simulink model "TremorStabilizingSimulation"  (Simulink 10.0)
settings: Solver=ode45  StartTime=0.0  StopTime=500  RelTol=1e-8  EnableMultiTasking=on
PreLoadFcn:
  | % Motor Parameters
  | 
  | J=0.01;     %kg*m^2
  | b=0.1;      %N*m/(rad/s)
  | K=0.01;     %V/(rad/s)
  | R=1;        %Ohm
  | L=0.5;      %H
libraries: simulink_extras x2, simulink x1
settings Model: Creator=deastman  LastModifiedBy=Aarranon
settings DataIOCC: LimitDataPoints=on  SignalLoggingSaveFormat=ModelDataLogs
settings OptimizationCC: ExpressionDepthLimit=2147483647  InitFltsAndDblsToZero=on
settings DebuggingCC: SolverPrmCheckMsg=warning  FcnCallInpInsideContextMsg=warning  StateNameClashWarn=warning
settings GRTTargetCC: GeneratePreprocessorConditionals=Disable all
settings ConfigComp: CovExternalEMLEnable=off

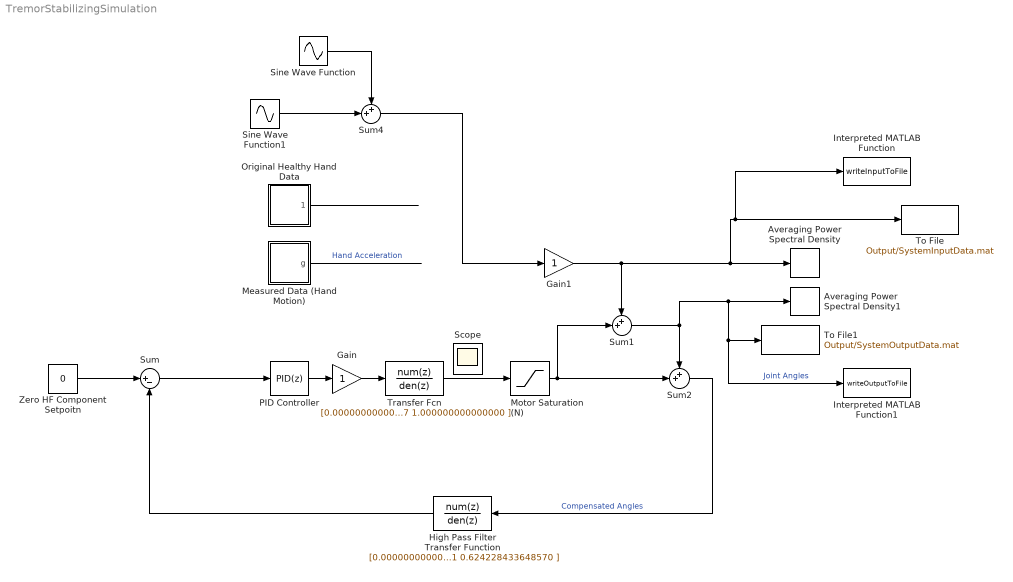
== system TremorStabilizingSimulation ==
  Averaging Power Spectral Density : simulink_extras/Additional Sinks/Averaging Power Spectral Density  npts=128  fftpts=512  HowOften=64  sampleT=2*1/104
      settings: SourceProductName=Simulink  SourceProductBaseCode=SL
  Averaging Power Spectral Density1 : simulink_extras/Additional Sinks/Averaging Power Spectral Density  npts=128  fftpts=512  HowOften=64  sampleT=2*1/104
      settings: SourceProductName=Simulink  SourceProductBaseCode=SL
  Gain : Gain
  Gain1 : Gain
  High Pass Filter Transfer Function : DiscreteTransferFcn  Numerator=[0.000000000000000 0.007900812829378 -0.007900812829378 ]  Denominator=[1.000000000000000 -1.580162565875511 0.624228433648570 ]  SampleTime=0.0100000000000000002  mask(DiscretizedDiscreteTransferFcn){}
      mask init:
      | %zoh
  Interpreted MATLAB Function : MATLABFcn  MATLABFcn=writeInputToFile  OutputDimensions=0
  Interpreted MATLAB Function1 : MATLABFcn  MATLABFcn=writeOutputToFile  OutputDimensions=0
  Measured Data (Hand Motion) : Subsystem
  Motor Saturation (N) : Saturate  UpperLimit=5.5/0.46  LowerLimit=-5.5/0.46
  "Original Healthy Hand Data " : Subsystem
  PID Controller : simulink/Continuous/PID Controller  Controller=PID  Form=Parallel  TimeDomain=Discrete-time  SampleTime=0.0100000000000000002  IntegratorMethod=Forward Euler  FilterMethod=Forward Euler  ControllerParametersSource=internal  P=25.000000000000000  I=0.000000000000000  D=26.270829861937610  UseFilter=on  N=9.516258196404047  TunerSelectOption=Frequency Response Based  InitialConditionSource=internal  InitialConditionForIntegrator=0  InitialConditionForFilter=0  DifferentiatorICPrevScaledInput=0  ExternalReset=none  TrackingMode=off  Kt=1  LimitOutput=off  UpperSaturationLimit=inf  LowerSaturationLimit=-inf  LinearizeAsGain=on  AntiWindupMode=none  Kb=1  POutMin=[]  POutMax=[]  IOutMin=[]  IOutMax=[]  DOutMin=[]  DOutMax=[]  NOutMin=[]  NOutMax=[]  SumOutMin=[]  SumOutMax=[]  SaturationOutMin=[]  SaturationOutMax=[]  PParamMin=[]  PParamMax=[]  IParamMin=[]  IParamMax=[]  DParamMin=[]  DParamMax=[]  NParamMin=[]  NParamMax=[]  KbParamMin=[]  KbParamMax=[]  KtParamMin=[]  KtParamMax=[]  KbOutMin=[]  KbOutMax=[]  KtOutMin=[]  KtOutMax=[]  IntegratorOutMin=[]  IntegratorOutMax=[]  FilterOutMin=[]  FilterOutMax=[]  SumI1OutMin=[]  SumI1OutMax=[]  SumI2OutMin=[]  SumI2OutMax=[]  SumI3OutMin=[]  SumI3OutMax=[]  SumI4OutMin=[]  SumI4OutMax=[]  SumDOutMin=[]  SumDOutMax=[]  DifferentiatorOutMin=[]  DifferentiatorOutMax=[]  FilterDiffOutCoefMin=[]  FilterDiffOutCoefMax=[]  ReciprocalOutMin=[]  ReciprocalOutMax=[]  SumDenOutMin=[]  SumDenOutMax=[]  SumNumOutMin=[]  SumNumOutMax=[]  DivideOutMin=[]  DivideOutMax=[]  IntegratorContinuousStateAttributes=''  IntegratorStateMustResolveToSignalObject=off  IntegratorRTWStateStorageClass=Auto  FilterContinuousStateAttributes=''  FilterStateMustResolveToSignalObject=off  FilterRTWStateStorageClass=Auto  ParallelPVariant=InternalParameters  IdealPVariant=Disabled  IVariant=InternalParameters  DVariant=InternalParameters  IntegratorVariant=Discrete  SatVariant=Disabled  AWVariant=Passthrough  PCopyVariant=Disabled  TRVariant=Disabled  FdbkBlocksVariant=Forward  IdealPFdbkVariant=Disabled  SatFdbkVariant=Disabled  DerivativeFilterVariant=ForwardEulerFilter  NVariant=InternalParameters  NCopyVariant=Disabled  FilterICVariant=InternalICsFilter  IntegratorICVariant=InternalICs  ExternalResetVariant=Disabled  TRSumVariant=Passthrough  SumFdbkVariant=Disabled  SumVariant=Sum_PID
  Sine Wave Function : Sin  Frequency=10*pi  Phase=54  SampleTime=0.0100000000000000002  mask(DiscretizedSource){}
      mask init:
      | %zoh
  Sine Wave Function1 : Sin  Frequency=2*2*pi  SampleTime=0.0100000000000000002  mask(DiscretizedSource){}
      mask init:
      | %zoh
  Sum : Sum  Inputs=|+-
  Sum1 : Sum  Inputs=++|
  Sum2 : Sum  Inputs=++|
  Sum4 : Sum  Inputs=++|
  To File : ToFile  Filename=Output/SystemInputData.mat  MatrixName=data  SaveFormat=Timeseries
  To File1 : ToFile  Filename=Output/SystemOutputData.mat  MatrixName=data  SaveFormat=Timeseries
  Transfer Fcn : DiscreteTransferFcn  Numerator=[0.000000000000000 0.009836316430835 -0.009836316430835 ]  Denominator=[1.000000000000000 -1.902113032590307 1.000000000000000 ]  SampleTime=0.0100000000000000002  mask(DiscretizedDiscreteTransferFcn){}
      mask init:
      | %zoh
  Zero HF Component Setpoitn : Constant  Value=0
  Scope : Scope
  wires:
  Zero HF Component Setpoitn/1 -> Sum/1
  High Pass Filter Transfer Function/1 -> Sum/2
  Sum2/1 -> High Pass Filter Transfer Function/1  "Compensated Angles"
  Motor Saturation (N)/1 -> Sum1/2, Sum2/2
  Sum1/1 -> Interpreted MATLAB Function1/1, To File1/1, Averaging Power Spectral Density1/1, Sum2/1  "Joint Angles"
  Sum/1 -> PID Controller/1
  Sine Wave Function/1 -> Sum4/1
  Sine Wave Function1/1 -> Sum4/2
  Gain1/1 -> Interpreted MATLAB Function/1, To File/1, Averaging Power Spectral Density/1, Sum1/1
  Transfer Fcn/1 -> Motor Saturation (N)/1
  "Original Healthy Hand Data "/1(Speed) -> ?
  PID Controller/1 -> Gain/1
  Gain/1 -> Transfer Fcn/1
  Sum4/1 -> Gain1/1
  Measured Data (Hand Motion)/1(g) -> ?  "Hand Acceleration"

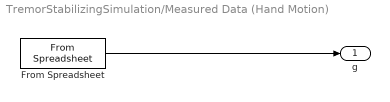
== system TremorStabilizingSimulation/Measured Data (Hand Motion) ==
  From Spreadsheet : FromSpreadsheet  FileName=\tremorx.csv  SheetName=tremorx  TreatFirstColumnAs=Data  SampleTime=1/104
  g : Outport
  wires:
  From Spreadsheet/1 -> g/1

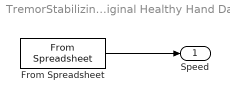
== system TremorStabilizingSimulation/Original Healthy Hand Data  ==
  From Spreadsheet : FromSpreadsheet  FileName=\origx.csv  SheetName=origx  TreatFirstColumnAs=Data  SampleTime=1/104
  Speed : Outport
  wires:
  From Spreadsheet/1 -> Speed/1
